simulink model "balancing_controller"  (R2015b)
settings: Solver=FixedStepDiscrete  StartTime=0.0  StopTime=tstop  FixedStep=T  RelTol=1e-3
values from neighbouring files (symbols this model uses):
  Ad = ss_disc.A    [balance_setup.m]    (also in swingup_setup.m)
  alpha_cal = -(360/4096) * (pi/180)    (= -0.00153398078789)    [balance_setup.m]    (also in swingup_setup.m)
  Bd = ss_disc.B    [balance_setup.m]    (also in swingup_setup.m)
  Cd = ss_disc.C    [balance_setup.m]    (also in swingup_setup.m)
  Dd = ss_disc.D    [balance_setup.m]    (also in swingup_setup.m)
  T = 0.001    [balance_setup.m]    (also in swingup_setup.m)
  theta_cal = -(360/4096) * (pi/180)    (= -0.00153398078789)    [balance_setup.m]    (also in swingup_setup.m)
  theta_freq = 4    [balance_setup.m]    (also in swingup_setup.m = 0)
  theta_ref = 0 * 45/180 * pi    (= 0)    [balance_setup.m]    (also in swingup_setup.m)
undefined symbols (not defined in the file or in its folder): Discrete, HIL, K_lqr, Time
libraries: quarc_library x4, ctrlSharedLib x1
settings Model: SimulationMode=external  ExtModeTrigType=signal  ExtModeTrigDuration=200000  ExtModeTrigDirection=either  ExtModeTrigLevel=0.500000  Creator=shadar  LastModifiedBy=maxcrisafulli
settings SolverCC: PositivePriorityOrder=on
settings RTWCC: SystemTargetFile=quarc_win64.tlc  TemplateMakefile=quarc_default_tmf  Description=QUARC Win64 Target
settings STFCustomTargetCC: GeneratePreprocessorConditionals=Use local settings  CPPClassGenCompliant=off
settings GRTTargetCC: ParMdlRefBuildCompliant=off  CompOptLevelCompliant=off  CombineOutputUpdateFcns=off  MatFileLogging=off  CPPClassGenCompliant=off  GRTInterface=on  UseToolchainInfoCompliant=off  ExtMode=on  ExtModeMexFile=quarc_comm

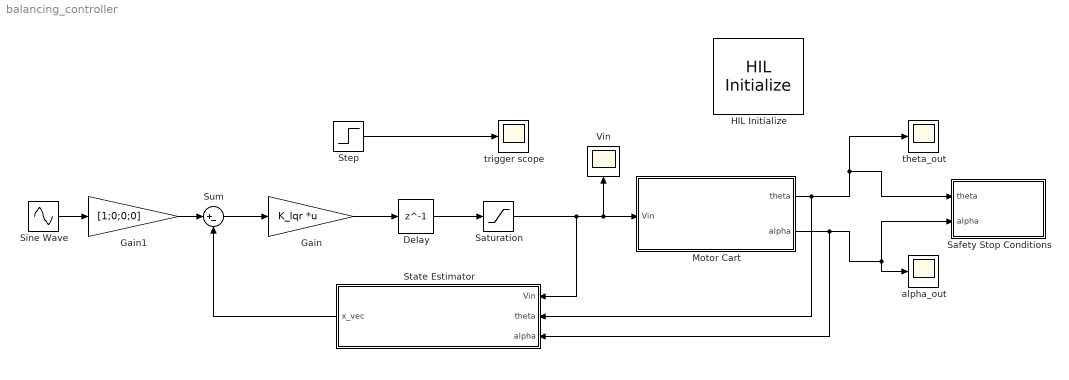
== system balancing_controller ==
  Delay : Delay  DelayLength=1  InitialCondition=0
  Gain : Gain  Gain=K_lqr  Multiplication=Matrix(K*u)
  Gain1 : Gain  Gain=[1;0;0;0]
  HIL Initialize : quarc_library/Data Acquisition/Generic/Configuration/HIL Initialize  object_name=HIL-1  board_type=q4  board_number=0  board_options=""  exclusive=off  active=on  hardware_clocks=[0:1]  clock_modes=[0 0]  initial_clock_frequencies=[]  set_clock_params_at_start=on  set_clock_params_at_switch_in=off  set_clock_frequencies_at_start=off  set_clock_frequencies_at_switch_in=off  analog_input_channels=[0:3]  analog_input_configurations=[]  analog_input_maximums=10  analog_input_minimums=-10  set_analog_input_params_at_start=off  set_analog_input_params_at_switch_in=off  analog_output_channels=[0:3]  analog_output_maximums=[10]  analog_output_minimums=[-10]  initial_analog_outputs=[0]  final_analog_outputs=[0]  watchdog_analog_outputs=0  set_analog_output_params_at_start=on  set_analog_output_params_at_switch_in=off  set_analog_outputs_at_start=on  set_analog_outputs_at_switch_in=off  set_analog_outputs_at_terminate=on  set_analog_outputs_at_switch_out=off  set_analog_outputs_on_watchdog=off  digital_input_channels=[]  digital_output_channels=[]  digital_output_configuration=[]  initial_digital_outputs=[1]  final_digital_outputs=[1]  watchdog_digital_outputs=[2]  set_digital_output_params_at_start=off  set_digital_output_params_at_switch_in=off  set_digital_outputs_at_start=on  set_digital_outputs_at_switch_in=off  set_digital_outputs_at_terminate=on  set_digital_outputs_at_switch_out=off  set_digital_outputs_on_watchdog=off  encoder_channels=[0:3]  quadrature=[4]  encoder_filter_frequency=(1/60e-9)/1  initial_encoder_counts=[0]  set_encoder_params_at_start=on  set_encoder_params_at_switch_in=off  set_encoder_counts_at_start=on  set_encoder_counts_at_switch_in=off  pwm_channels=[]  pwm_modes=[0]  pwm_frequency=(1/60e-9)/1024  pwm_configuration=[]  pwm_alignment=[]  pwm_polarity=[]  pwm_leading_deadband=[]  pwm_trailing_deadband=[]  initial_pwm_outputs=[0]  final_pwm_outputs=[0]  watchdog_pwm_outputs=[]  set_pwm_params_at_start=on  set_pwm_params_at_switch_in=off  set_pwm_outputs_at_start=on  set_pwm_outputs_at_switch_in=off  set_pwm_outputs_at_terminate=on  set_pwm_outputs_at_switch_out=off  set_pwm_outputs_on_watchdog=off  other_output_channels=[]  initial_other_outputs=[]  final_other_outputs=[]  watchdog_other_outputs=[]  set_other_outputs_at_start=off  set_other_outputs_at_switch_in=off  set_other_outputs_at_terminate=off  set_other_outputs_at_switch_out=off  set_other_outputs_on_watchdog=off
  "Motor Cart " : Subsystem
  Safety Stop Conditions : Subsystem
  Saturation : Saturate  UpperLimit=10  LowerLimit=-10
  Sine Wave : Sin  Amplitude=theta_ref  Frequency=theta_freq  SampleTime=T
  State Estimator : Subsystem
  Step : Step  Time=0.001  SampleTime=0
  Sum : Sum  Inputs=|+-
  Vin : Scope
  "alpha_out " : Scope
  theta_out : Scope
  trigger scope : Scope
  wires:
  Step/1 -> trigger scope/1
  "Motor Cart "/1(theta) -> Safety Stop Conditions/1(theta), theta_out/1, State Estimator/2(theta)
  "Motor Cart "/2(alpha) -> State Estimator/3(alpha), Safety Stop Conditions/2(alpha), "alpha_out "/1
  State Estimator/1(x_vec) -> Sum/2
  Saturation/1 -> "Motor Cart "/1(Vin), Vin/1, State Estimator/1(Vin)
  Delay/1 -> Saturation/1
  Gain1/1 -> Sum/1
  Sine Wave/1 -> Gain1/1
  Sum/1 -> Gain/1
  Gain/1 -> Delay/1

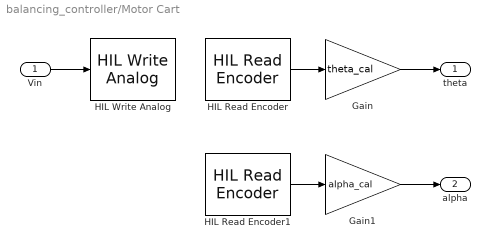
== system balancing_controller/Motor Cart  ==
  Vin : Inport
  Gain : Gain  Gain=theta_cal
  Gain1 : Gain  Gain=alpha_cal
  HIL Read Encoder : quarc_library/Data Acquisition/Generic/Immediate I//O/HIL Read Encoder  object_name=HIL-1  channels=0  sample_time=T  active=on  vector_output=on  data_type_mode=Inherit via back propagation  data_type=double
  HIL Read Encoder1 : quarc_library/Data Acquisition/Generic/Immediate I//O/HIL Read Encoder  object_name=HIL-1  channels=2  sample_time=qc_get_step_size  active=on  vector_output=off  data_type_mode=Inherit via back propagation  data_type=double
  HIL Write Analog : quarc_library/Data Acquisition/Generic/Immediate I//O/HIL Write Analog  object_name=HIL-1  channels=0  sample_time=T  active=off  vector_input=off
  theta : Outport
  alpha : Outport  Port=2
  wires:
  Vin/1 -> HIL Write Analog/1
  HIL Read Encoder/1 -> Gain/1
  Gain/1 -> theta/1
  HIL Read Encoder1/1 -> Gain1/1
  Gain1/1 -> alpha/1

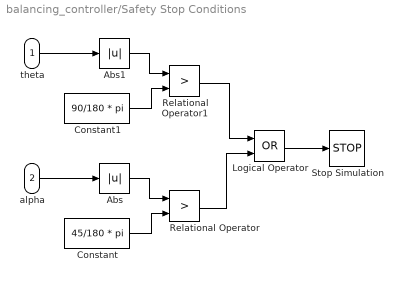
== system balancing_controller/Safety Stop Conditions ==
  theta : Inport
  alpha : Inport  Port=2
  Abs : Abs
  Abs1 : Abs
  Constant : Constant  Value=45/180 * pi
  Constant1 : Constant  Value=90/180 * pi
  Logical Operator : Logic  Operator=OR  AllPortsSameDT=off  OutDataTypeStr=boolean
  Relational Operator : RelationalOperator  Operator=>  OutDataTypeStr=boolean
  Relational Operator1 : RelationalOperator  Operator=>  OutDataTypeStr=boolean
  Stop Simulation : Stop
  wires:
  Abs/1 -> Relational Operator/1
  Constant/1 -> Relational Operator/2
  alpha/1 -> Abs/1
  theta/1 -> Abs1/1
  Relational Operator/1 -> Logical Operator/2
  Relational Operator1/1 -> Logical Operator/1
  Abs1/1 -> Relational Operator1/1
  Constant1/1 -> Relational Operator1/2
  Logical Operator/1 -> Stop Simulation/1

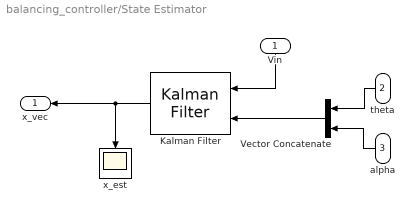
== system balancing_controller/State Estimator ==
  Vin : Inport
  theta : Inport  Port=2
  alpha : Inport  Port=3
  Kalman Filter : ctrlSharedLib/Kalman Filter  TimeDomain=Discrete-Time  UseCurrentEstimator=on  ModelSource=Individual A, B, C, D matrices  ModelSourceVariable=ss(0.95,1,1,0,1)  A=Ad  B=Bd  C=Cd  D=Dd  NumberOfStates=1  NumberOfInputs=1  NumberOfOutputs=1  InitialEstimateSource=Dialog  X0=0  P0=10  UseK=off  UseGH=off  NumberOfProcessNoiseInputs=1  G=1  TimeInvariantG=on  H=0  TimeInvariantH=on  Q=1  TimeInvariantQ=on  R=100  TimeInvariantR=on  N=0  TimeInvariantN=on  AddInputPort=on  AddEnablePort=off  OutputEstimatedY=off  OutputP=off  Ts=T
  Vector Concatenate : Concatenate
  x_est : Scope
  x_vec : Outport
  wires:
  alpha/1 -> Vector Concatenate/2
  theta/1 -> Vector Concatenate/1
  Vin/1 -> Kalman Filter/1
  Vector Concatenate/1 -> Kalman Filter/2
  Kalman Filter/1 -> x_vec/1, x_est/1
